simulink model "gm_uz_endat_interface_2025b"  (R2025b)
settings: Solver=FixedStepDiscrete  StartTime=0.0  StopTime=1.3e-3  RelTol=1e-3
undefined symbols (not defined in the file or in its folder): binary_or_gray, bit_sum, delay_first_clk_on_off, endat_clk_divider, endat_encoder_bit_width_multi_turn, endat_encoder_bit_width_single_turn, endat_encoder_number_of_CRC_bits, f_ADC, f_clock, PLL, t_ADC, t_clock, XData
libraries: hdlmdlgenlib x123, simulink x35, hdlsllib x29, simulink_extras x13
(part 2 of 4)

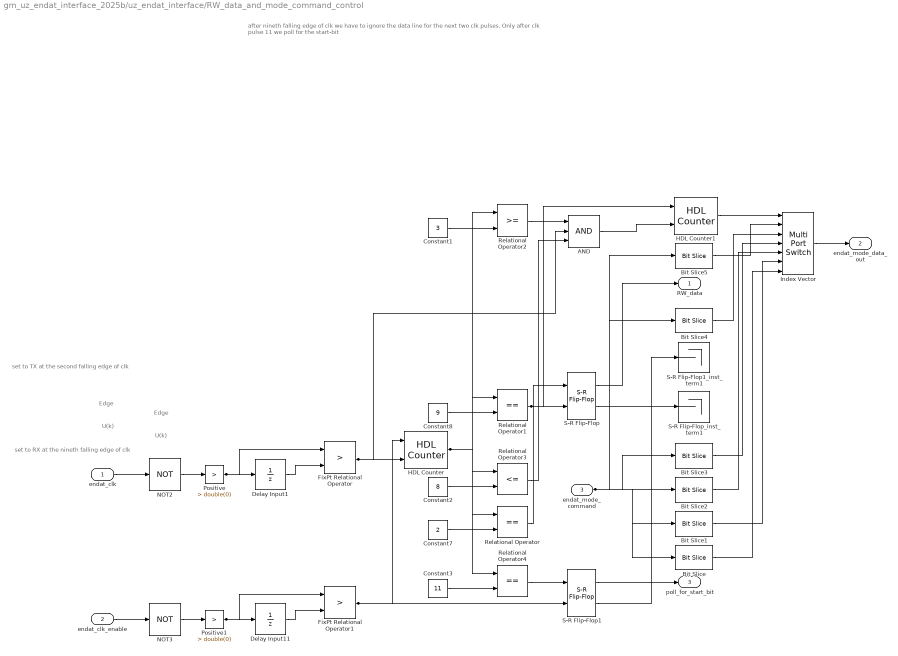
== system gm_uz_endat_interface_2025b/uz_endat_interface/RW_data_and_mode_command_control ==
  note: U(k)
  note: Edge
  note: U(k)
  note: Edge
  note: after nineth falling edge of clk we have to ignore the data line for the next two clk pulses. Only after clk pulse 11 we poll for the start-bit
  note: set to RX at the nineth falling edge of clk
  note: set to TX at the second falling edge of clk
  endat_clk : Inport  OutDataTypeStr=boolean  PortDimensions=1  SampleTime=1e-08
  endat_clk_enable : Inport  Port=2  OutDataTypeStr=boolean  PortDimensions=1  SampleTime=1e-08
  endat_mode_command : Inport  Port=3  OutDataTypeStr=uint32  PortDimensions=1  SampleTime=1e-08
  AND : Logic  Inputs=3  AllPortsSameDT=off  OutDataTypeStr=boolean  SampleTime=1e-08
  Bit Slice : hdlsllib/Logic and Bit Operations/Bit Slice  lidx=double(0)  ridx=double(0)
  Bit Slice1 : hdlsllib/Logic and Bit Operations/Bit Slice  lidx=double(1)  ridx=double(1)
  Bit Slice2 : hdlsllib/Logic and Bit Operations/Bit Slice  lidx=double(2)  ridx=double(2)
  Bit Slice3 : hdlsllib/Logic and Bit Operations/Bit Slice  lidx=double(3)  ridx=double(3)
  Bit Slice4 : hdlsllib/Logic and Bit Operations/Bit Slice  lidx=double(4)  ridx=double(4)
  Bit Slice5 : hdlsllib/Logic and Bit Operations/Bit Slice  lidx=double(5)  ridx=double(5)
  Constant1 : Constant  Value=3  OutDataTypeStr=uint8  SampleTime=1e-08
  Constant2 : Constant  Value=8  OutDataTypeStr=uint8  SampleTime=1e-08
  Constant3 : Constant  Value=11  OutDataTypeStr=uint8  SampleTime=1e-08
  Constant7 : Constant  Value=2  OutDataTypeStr=uint8  SampleTime=1e-08
  Constant8 : Constant  Value=9  OutDataTypeStr=uint8  SampleTime=1e-08
  Delay Input1 : UnitDelay  SampleTime=1e-08
  Delay Input11 : UnitDelay  SampleTime=1e-08
  FixPt Relational Operator : RelationalOperator  Operator=>  OutDataTypeStr=boolean  SampleTime=1e-08  InputSameDT=off
  FixPt Relational Operator1 : RelationalOperator  Operator=>  OutDataTypeStr=boolean  SampleTime=1e-08  InputSameDT=off
  HDL Counter : hdlsllib/Sources/HDL Counter  CountType=Free running  CountInit=0  CountStep=1  CountMax=25  CountFromType=Initial value  CountFrom=0  CountResetPort=on  CountLoadPort=off  CountEnbPort=on  CountDirPort=off  CountHitOutputPort=off  CountDataType=Unsigned  CountWordLen=8  CountFracLen=0  CountSampTime=1
  HDL Counter1 : hdlsllib/Sources/HDL Counter  CountType=Count limited  CountInit=0  CountStep=1  CountMax=5  CountFromType=Initial value  CountFrom=0  CountResetPort=on  CountLoadPort=off  CountEnbPort=on  CountDirPort=off  CountHitOutputPort=off  CountDataType=Unsigned  CountWordLen=8  CountFracLen=0  CountSampTime=1
  Index Vector : MultiPortSwitch  DataPortOrder=Zero-based contiguous  Inputs=6  DiagnosticForDefault=None  zeroidx=on  OutDataTypeStr=fixdt(0, 1, 0)  SampleTime=1e-08  SaturateOnIntegerOverflow=off  InputSameDT=off
  NOT2 : Logic  Operator=NOT  Inputs=1  AllPortsSameDT=off  OutDataTypeStr=boolean  SampleTime=1e-08
  NOT3 : Logic  Operator=NOT  Inputs=1  AllPortsSameDT=off  OutDataTypeStr=boolean  SampleTime=1e-08
  Positive : simulink/Logic and Bit Operations/Compare To Constant  relop=>  const=double(0)  OutDataTypeStr=boolean
  Positive1 : simulink/Logic and Bit Operations/Compare To Constant  relop=>  const=double(0)  OutDataTypeStr=boolean
  Relational Operator : RelationalOperator  Operator===  OutDataTypeStr=boolean  SampleTime=1e-08  InputSameDT=off
  Relational Operator1 : RelationalOperator  Operator===  OutDataTypeStr=boolean  SampleTime=1e-08  InputSameDT=off
  Relational Operator2 : RelationalOperator  OutDataTypeStr=boolean  SampleTime=1e-08  InputSameDT=off
  Relational Operator3 : RelationalOperator  Operator=<=  OutDataTypeStr=boolean  SampleTime=1e-08  InputSameDT=off
  Relational Operator4 : RelationalOperator  Operator===  OutDataTypeStr=boolean  SampleTime=1e-08  InputSameDT=off
  S-R Flip-Flop : simulink_extras/Flip Flops/S-R Flip-Flop  initial_condition=0
  S-R Flip-Flop1 : simulink_extras/Flip Flops/S-R Flip-Flop  initial_condition=0
  S-R Flip-Flop1_inst_term1 : Terminator
  S-R Flip-Flop_inst_term1 : Terminator
  RW_data : Outport  SampleTime=1e-08
  endat_mode_data_out : Outport  Port=2  SampleTime=1e-08
  poll_for_start_bit : Outport  Port=3  SampleTime=1e-08
  wires:
  endat_clk/1 -> NOT2/1
  Positive1/1 -> FixPt Relational Operator1/1, Delay Input11/1
  Bit Slice3/1 -> Index Vector/4
  endat_clk_enable/1 -> NOT3/1
  Delay Input1/1 -> FixPt Relational Operator/2
  NOT2/1 -> Positive/1
  Delay Input11/1 -> FixPt Relational Operator1/2
  NOT3/1 -> Positive1/1
  Positive/1 -> FixPt Relational Operator/1, Delay Input1/1
  FixPt Relational Operator/1 -> AND/2, HDL Counter/2
  FixPt Relational Operator1/1 -> S-R Flip-Flop1/2, HDL Counter/1
  Bit Slice4/1 -> Index Vector/3
  Constant1/1 -> Relational Operator2/2
  Constant7/1 -> Relational Operator/2
  Constant8/1 -> Relational Operator1/2
  HDL Counter/1 -> Relational Operator4/1, Relational Operator3/1, Relational Operator1/1, Relational Operator2/1, Relational Operator/1
  Constant3/1 -> Relational Operator4/2
  Constant2/1 -> Relational Operator3/2
  Relational Operator2/1 -> AND/1
  Relational Operator1/1 -> S-R Flip-Flop/2, HDL Counter1/1
  Relational Operator3/1 -> AND/3
  Relational Operator/1 -> S-R Flip-Flop/1
  Relational Operator4/1 -> S-R Flip-Flop1/1
  S-R Flip-Flop/2 -> S-R Flip-Flop_inst_term1/1
  S-R Flip-Flop/1 -> RW_data/1
  AND/1 -> HDL Counter1/2
  endat_mode_command/1 -> Bit Slice4/1, Bit Slice3/1, Bit Slice5/1, Bit Slice2/1, Bit Slice1/1, Bit Slice/1
  S-R Flip-Flop1/1 -> poll_for_start_bit/1
  S-R Flip-Flop1/2 -> S-R Flip-Flop1_inst_term1/1
  Index Vector/1 -> endat_mode_data_out/1
  HDL Counter1/1 -> Index Vector/1
  Bit Slice5/1 -> Index Vector/2
  Bit Slice2/1 -> Index Vector/5
  Bit Slice1/1 -> Index Vector/6
  Bit Slice/1 -> Index Vector/7

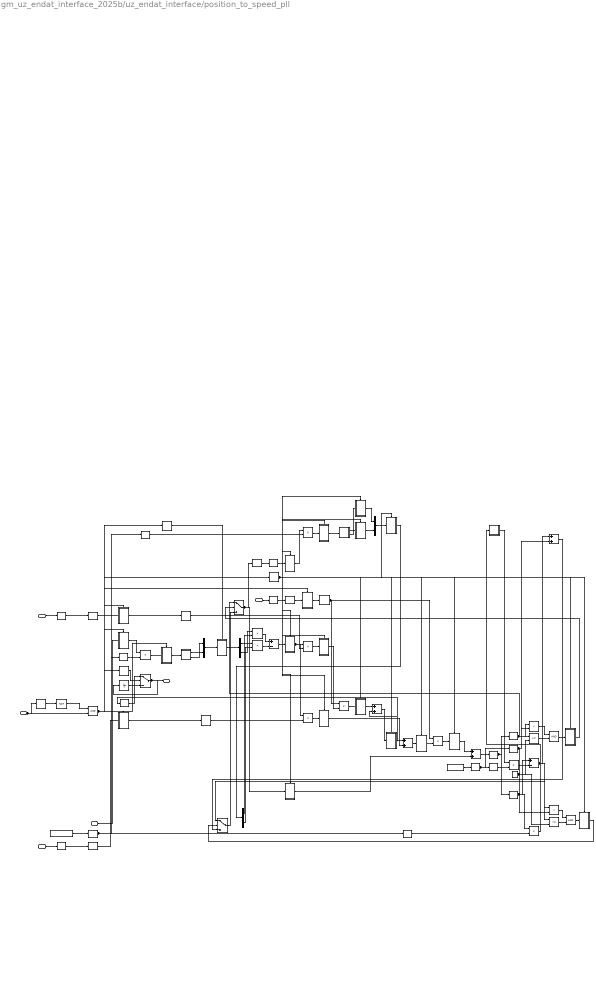
== system gm_uz_endat_interface_2025b/uz_endat_interface/position_to_speed_pll ==
  note: pi_controller
  note: +/- 198000
  note: -2 ... 2
  note: wrap 2pi
  note: <<1
  note: phase discriminator
  note: -1 ... 1
  note: pll
  note: -1 ... 1
  note: integrator
  note: 20
  note: +/- 1300
  note: remainder
  position_mech_SI : Inport  OutDataTypeStr=fixdt(0, 27, 24)  PortDimensions=1  SampleTime=1e-08
  t_sample : Inport  Port=2  OutDataTypeStr=fixdt(0, 18, 24)  PortDimensions=1  SampleTime=1e-08
  kp_pll : Inport  Port=3  OutDataTypeStr=fixdt(0, 18, 5)  PortDimensions=1  SampleTime=1e-08
  ki_pll : Inport  Port=4  OutDataTypeStr=fixdt(0, 18, 0)  PortDimensions=1  SampleTime=1e-08
  Trigger : Inport  Port=5  OutDataTypeStr=boolean  SampleTime=1e-08
  AND : Logic  AllPortsSameDT=off  OutDataTypeStr=boolean  SampleTime=1e-08
  AND1 : Logic  AllPortsSameDT=off  OutDataTypeStr=boolean  SampleTime=1e-08
  Constant1 : Constant  Value=0.1591548919677734375  OutDataTypeStr=fixdt(0, 18, 20)  SampleTime=1e-08
  Constant7 : Constant  Value=0  OutDataTypeStr=fixdt(0, 27, 24)  SampleTime=1e-08
  Constant8 : Constant  Value=6.283172607421875  OutDataTypeStr=fixdt(0, 18, 15)  SampleTime=1e-08
  Delay : Subsystem
      settings: MinAlgLoopOccurrences=on
  Delay1 : Subsystem
      settings: MinAlgLoopOccurrences=on
  Delay10 : Subsystem
      settings: MinAlgLoopOccurrences=on
  Delay11 : Subsystem
      settings: MinAlgLoopOccurrences=on
  Delay12 : Subsystem
      settings: MinAlgLoopOccurrences=on
  Delay13 : Subsystem
      settings: MinAlgLoopOccurrences=on
  Delay14 : Subsystem
      settings: MinAlgLoopOccurrences=on
  Delay18 : Subsystem
      settings: MinAlgLoopOccurrences=on
  Delay19 : Subsystem
      settings: MinAlgLoopOccurrences=on
  Delay2 : Subsystem
      settings: MinAlgLoopOccurrences=on
  Delay20 : Subsystem
      settings: MinAlgLoopOccurrences=on
  Delay21 : Subsystem
      settings: MinAlgLoopOccurrences=on
  Delay22 : Subsystem
      settings: MinAlgLoopOccurrences=on
  Delay23 : Subsystem
      settings: MinAlgLoopOccurrences=on
  Delay3 : Subsystem
      settings: MinAlgLoopOccurrences=on
  Delay4 : Subsystem
      settings: MinAlgLoopOccurrences=on
  Delay5 : Subsystem
      settings: MinAlgLoopOccurrences=on
  Delay6 : Subsystem
      settings: MinAlgLoopOccurrences=on
  Delay7 : Subsystem
      settings: MinAlgLoopOccurrences=on
  Delay8 : Subsystem
      settings: MinAlgLoopOccurrences=on
  Delay9 : Subsystem
      settings: MinAlgLoopOccurrences=on
  From{,1..6,11,13..15} (11 alike) : hdlmdlgenlib/Buffer
  Goto{,1..3,8,10..11} (7 alike) : hdlmdlgenlib/Buffer
  Product1 : Product  Inputs=**  OutDataTypeStr=fixdt(1, 27, 23)  SampleTime=1e-08
  Product10 : Product  Inputs=**  OutDataTypeStr=fixdt(1, 27, 20)  SampleTime=1e-08
  Product2 : Product  Inputs=**  OutDataTypeStr=fixdt(1, 27, 25)  SampleTime=1e-08
  Product3 : Product  Inputs=**  OutDataTypeStr=fixdt(1, 27, 25)  SampleTime=1e-08
  Product4 : Product  Inputs=**  OutDataTypeStr=fixdt(1, 27, 20)  SampleTime=1e-08
  Product5 : Product  Inputs=**  OutDataTypeStr=fixdt(1, 27, 8)  SampleTime=1e-08
  Product6 : Product  Inputs=**  OutDataTypeStr=fixdt(1, 27, 14)  SampleTime=1e-08
  Product7 : Product  Inputs=**  OutDataTypeStr=fixdt(1, 27, 23)  SampleTime=1e-08
  Product8 : Product  Inputs=**  OutDataTypeStr=fixdt(1, 27, 26)  SampleTime=1e-08
  Product9 : Product  Inputs=**  OutDataTypeStr=fixdt(1, 27, 20)  SampleTime=1e-08
  Relational Operator1 : RelationalOperator  Operator=<  OutDataTypeStr=boolean  SampleTime=1e-08  InputSameDT=off
  Relational Operator2 : RelationalOperator  OutDataTypeStr=boolean  SampleTime=1e-08  InputSameDT=off
  Relational Operator3 : RelationalOperator  Operator=<  OutDataTypeStr=boolean  SampleTime=1e-08  InputSameDT=off
  Relational Operator4 : RelationalOperator  OutDataTypeStr=boolean  SampleTime=1e-08  InputSameDT=off
  Sine HDL Optimized : Subsystem  mask(Sine and Cosine HDL optimized block){OutputFormula=sin(2*pi*u) and cos(2*pi*u), NumDataPoints=double(256), TableDataTypeStr=fixdt(0,26,20), SimulateLUTROMDelay=off}
      mask prompts: OutputFormula "Simulink:masks:OutputFormula_MP"; NumDataPoints "HDLShared:hdlshared:CosineHDL_Npts"; TableDataTypeStr "Simulink:blkprm_prompts:TABLE_UNIFIEDDATATYPE"; SimulateLUTROMDelay "HDLShared:hdlshared:CosineHDL_SimulateLUTDelay"
      mask help: Sine and Cosine HDL optimized block using quarter wave symmetry, and HDL friendly settings.
      mask init:
      | NumDataPoints = double(256);
      | OutputFormula = double(4);
      | SampleTime = double(-1);
      | SimulateLUTROMDelay = double(0);
      | TableDataTypeStr = fixdt(0,26,20);
      | curr_blk_name = 'uz_endat_interface_2025b/uz_endat_interface/position_to_speed_pll/Sine\nHDL Optimized';
      | sys_name = 'uz_endat_interface_2025b/uz_endat_interface/position_to_speed_pll';
      mask Help: helpview([docroot '/hdlcoder/helptargets.map'],'SineAndCosineHDL_Optimized');
      mask TypeOptions OutputFormula: sin(2*pi*u) | cos(2*pi*u) | exp(j*2*pi*u) | sin(2*pi*u) and cos(2*pi*u)
      mask Display:
      | port_label('input',1,'u')
      | port_label('output',1,'sin(2*pi*u)')
      | port_label('output',2,'cos(2*pi*u)')
      | xpos = 0.35;
      | yoffset = 0.5;
      | if ( SimulateLUTROMDelay )
      |   text(xpos,yoffset,'HDL (Z^{-1})','texmode','on')
      | else
      |    text(xpos,yoffset,'HDL')
      | end
  Sine HDL Optimized1 : Subsystem  mask(Sine and Cosine HDL optimized block){OutputFormula=sin(2*pi*u) and cos(2*pi*u), NumDataPoints=double(256), TableDataTypeStr=fixdt(0,26,20), SimulateLUTROMDelay=off}
      mask prompts: OutputFormula "Simulink:masks:OutputFormula_MP"; NumDataPoints "HDLShared:hdlshared:CosineHDL_Npts"; TableDataTypeStr "Simulink:blkprm_prompts:TABLE_UNIFIEDDATATYPE"; SimulateLUTROMDelay "HDLShared:hdlshared:CosineHDL_SimulateLUTDelay"
      mask help: Sine and Cosine HDL optimized block using quarter wave symmetry, and HDL friendly settings.
      mask init:
      | NumDataPoints = double(256);
      | OutputFormula = double(4);
      | SampleTime = double(-1);
      | SimulateLUTROMDelay = double(0);
      | TableDataTypeStr = fixdt(0,26,20);
      | curr_blk_name = 'uz_endat_interface_2025b/uz_endat_interface/position_to_speed_pll/Sine\nHDL Optimized1';
      | sys_name = 'uz_endat_interface_2025b/uz_endat_interface/position_to_speed_pll';
      mask Help: helpview([docroot '/hdlcoder/helptargets.map'],'SineAndCosineHDL_Optimized');
      mask TypeOptions OutputFormula: sin(2*pi*u) | cos(2*pi*u) | exp(j*2*pi*u) | sin(2*pi*u) and cos(2*pi*u)
      mask Display:
      | port_label('input',1,'u')
      | port_label('output',1,'sin(2*pi*u)')
      | port_label('output',2,'cos(2*pi*u)')
      | xpos = 0.35;
      | yoffset = 0.5;
      | if ( SimulateLUTROMDelay )
      |   text(xpos,yoffset,'HDL (Z^{-1})','texmode','on')
      | else
      |    text(xpos,yoffset,'HDL')
      | end
  Sum1 : Sum  Inputs=+-  OutDataTypeStr=fixdt(1, 27, 24)  AccumDataTypeStr=fixdt(1, 27, 24)  SampleTime=1e-08
  Sum2 : Sum  OutDataTypeStr=fixdt(1, 27, 16)  AccumDataTypeStr=fixdt(1, 32, 20)  SampleTime=1e-08
  Sum3 : Sum  OutDataTypeStr=fixdt(1, 27, 14)  AccumDataTypeStr=fixdt(1, 30, 16)  SampleTime=1e-08
  Sum4 : Sum  OutDataTypeStr=fixdt(1, 27, 23)  AccumDataTypeStr=fixdt(1, 31, 26)  SampleTime=1e-08
  Sum5 : Sum  Inputs=+-  OutDataTypeStr=fixdt(1, 27, 23)  AccumDataTypeStr=fixdt(1, 28, 23)  SampleTime=1e-08
  Sum6 : Sum  OutDataTypeStr=fixdt(1, 27, 23)  AccumDataTypeStr=fixdt(1, 28, 23)  SampleTime=1e-08
  Switch3 : Switch  Criteria=u2 > Threshold  Threshold="fi(0,0,1,0,\"hex\",\"0\")"  OutDataTypeStr=fixdt(1, 27, 23)  SampleTime=1e-08  SaturateOnIntegerOverflow=off  InputSameDT=off
  Switch4 : Switch  Criteria=u2 > Threshold  Threshold="fi(0,0,1,0,\"hex\",\"0\")"  OutDataTypeStr=fixdt(1, 27, 23)  SampleTime=1e-08  SaturateOnIntegerOverflow=off  InputSameDT=off
  Trigger_delay : Delay  DelayLength=double(1)  InitialCondition=0
  Trigger_delayed_inverted_and_Trigger : Logic  AllPortsSameDT=off  OutDataTypeStr=boolean  SampleTime=1e-08
  delayMatch{,1..5} (6 alike) : Delay  DelayLength=double(1)  InitialCondition=0
  fixed_point_floor : Subsystem
  mux : Mux  Inputs=2
  mux1 : Mux  Inputs=2
  not_Trigger_delayed : Logic  Operator=NOT  Inputs=1  AllPortsSameDT=off  OutDataTypeStr=boolean  SampleTime=1e-08
  omega_mechbypassMux : Switch  Criteria=u2 ~= 0  Threshold=double(0)  OutDataTypeStr=fixdt(1, 27, 16)  SampleTime=1e-08  SaturateOnIntegerOverflow=off  InputSameDT=off
  out0_bypass : UnitDelay  InitialCondition="fi(0,1,27,16,\"hex\",\"0000000\")"  SampleTime=1e-08
  t : Demux  Outputs=2
  t1 : Demux  Outputs=2
  t2 : hdlmdlgenlib/Buffer
  speed_mech_SI : Outport  SampleTime=1e-08  InitialOutput=[0]
  wires:
  Product5/1 -> Delay5/1(in0)
  delayMatch1/1 -> Delay2/Enable, Delay11/Enable, Delay9/Enable, Delay18/Enable, Delay5/Enable, Delay3/Enable, Delay21/Enable, Delay20/Enable, Delay12/Enable, Delay10/Enable, Delay/Enable, Delay4/Enable, Delay23/Enable, Delay19/Enable, Delay22/Enable
  Trigger/1 -> Trigger_delayed_inverted_and_Trigger/2, Trigger_delay/1
  Goto10/1 -> From15/1, From11/1
  Goto3/1 -> From5/1, From4/1, From6/1
  ki_pll/1 -> Goto2/1
  Goto1/1 -> From1/1
  Constant1/1 -> Goto3/1
  Trigger_delay/1 -> not_Trigger_delayed/1
  t_sample/1 -> Goto/1
  Sine HDL Optimized/2(y) -> Delay23/1(in0)
  delayMatch3/1 -> Product8/1, Product4/1
  Product6/1 -> Delay3/1(in0)
  Goto8/1 -> From3/1
  Delay6/1(out0) -> delayMatch3/1
  kp_pll/1 -> Goto1/1
  Delay11/1(out0) -> Product9/1
  Switch3/1 -> Goto8/1, Delay19/1(in0)
  omega_mechbypassMux/1 -> out0_bypass/1, speed_mech_SI/1
  Goto2/1 -> From2/1
  Product4/1 -> Delay4/1(in0)
  not_Trigger_delayed/1 -> Trigger_delayed_inverted_and_Trigger/1
  Delay12/1(out0) -> Sine HDL Optimized/1(u)
  From2/1 -> Delay7/1(in0)
  Goto/1 -> From/1
  Trigger_delayed_inverted_and_Trigger/1 -> Delay7/Enable, delayMatch1/1, Delay14/Enable, Delay13/Enable, Delay8/Enable, delayMatch/1, delayMatch5/1, Delay6/Enable
  position_mech_SI/1 -> Delay13/1(in0)
  From3/1 -> Delay11/1(in0)
  From1/1 -> Delay8/1(in0)
  Delay7/1(out0) -> delayMatch4/1
  Delay14/1(out0) -> Sine HDL Optimized1/1(u)
  Sine HDL Optimized1/1(x) -> mux/2
  Delay13/1(out0) -> Product10/1
  From6/1 -> Product10/2
  Delay1/1(out0) -> t/1
  delayMatch5/1 -> omega_mechbypassMux/2
  out0_bypass/1 -> omega_mechbypassMux/3
  t2/1 -> omega_mechbypassMux/1
  Delay8/1(out0) -> delayMatch2/1
  From5/1 -> Product9/2
  Product10/1 -> Delay14/1(in0)
  Delay4/1(out0) -> Sum2/1
  delayMatch/1 -> Delay1/Enable
  From15/1 -> Product7/1, Sum5/1
  Sine HDL Optimized/1(x) -> Delay22/1(in0)
  Sum1/1 -> Delay2/1(in0)
  delayMatch4/1 -> Product5/2
  Sine HDL Optimized1/2(y) -> mux/1
  From/1 -> Delay6/1(in0)
  Product2/1 -> Sum1/2
  mux/1 -> Delay1/1(in0)
  delayMatch2/1 -> Product6/2
  Switch4/1 -> Switch3/3
  Sum4/1 -> Goto10/1
  t/2 -> Product3/1
  t/1 -> Product2/1
  t1/2 -> Product2/2
  t1/1 -> Product3/2
  Product3/1 -> Sum1/1
  Delay2/1(out0) -> Product6/1, Product5/1
  AND1/1 -> Delay20/1(in0)
  Delay19/1(out0) -> Sum4/2
  Product9/1 -> Delay12/1(in0)
  Delay5/1(out0) -> Product4/2
  Delay3/1(out0) -> Sum3/2
  Delay23/1(out0) -> mux1/1
  Delay22/1(out0) -> mux1/2
  mux1/1 -> Delay18/1(in0)
  Sum2/1 -> Delay/1(in0)
  Delay18/1(out0) -> t1/1
  Delay/1(out0) -> t2/1, Sum2/2, Sum3/1
  Sum3/1 -> Delay9/1(in0)
  From4/1 -> Product7/2
  Delay9/1(out0) -> Product8/2
  Product8/1 -> Delay10/1(in0)
  From14/1 -> Product1/2
  Delay10/1(out0) -> Sum4/1
  Constant8/1 -> Goto11/1
  Goto11/1 -> From13/1, From14/1
  fixed_point_floor/1(y) -> Product1/1
  From11/1 -> Switch3/1, Relational Operator2/1, Relational Operator1/1
  From13/1 -> Relational Operator3/2, Sum6/2, Relational Operator1/2
  Product1/1 -> Sum5/2
  Constant7/1 -> Relational Operator4/2, Relational Operator2/2
  Relational Operator1/1 -> AND/1
  Relational Operator2/1 -> AND/2
  Sum5/1 -> Switch4/1, Sum6/1, Relational Operator4/1, Relational Operator3/1
  Product7/1 -> fixed_point_floor/1(x)
  Sum6/1 -> Switch4/3
  AND/1 -> Delay21/1(in0)
  Delay20/1(out0) -> Switch4/2
  Relational Operator3/1 -> AND1/1
  Relational Operator4/1 -> AND1/2
  Delay21/1(out0) -> Switch3/2

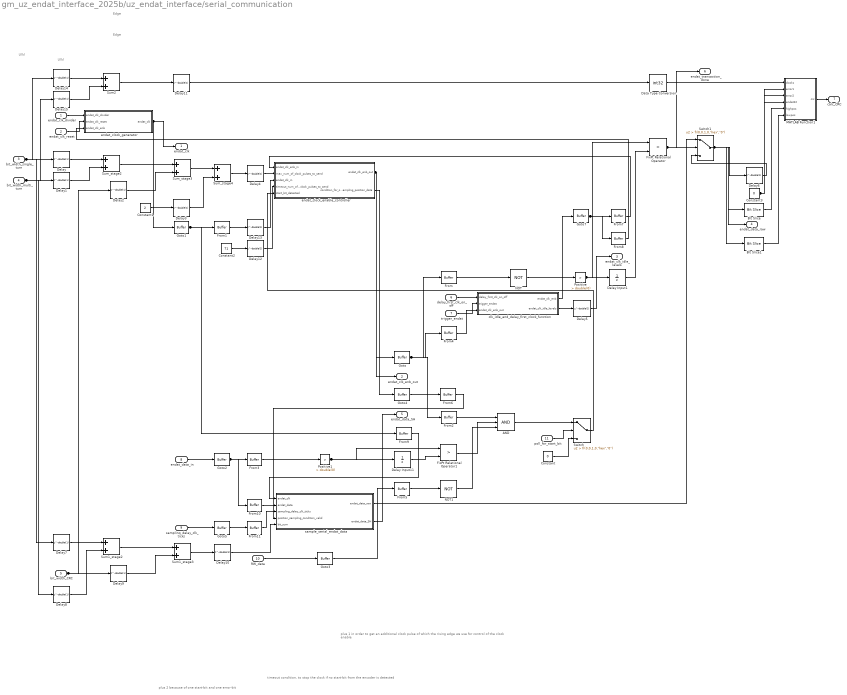
== system gm_uz_endat_interface_2025b/uz_endat_interface/serial_communication ==
  note: U(k)
  note: Edge
  note: U(k)
  note: Edge
  note: plus 1 in order to get an additional clock pulse of which the rising edge we use for control of the clock enable
  note: timeout condition, to stop the clock if no start-bit from the encoder is detected
  note: plus 2 because of one start-bit and one error-bit
  endat_clk_divider : Inport  OutDataTypeStr=uint32  PortDimensions=1  SampleTime=1e-08
  endat_clk_reset : Inport  Port=2  OutDataTypeStr=boolean  PortDimensions=1  SampleTime=1e-08
  bit_width_single_turn : Inport  Port=3  OutDataTypeStr=uint32  PortDimensions=1  SampleTime=1e-08
  bit_width_multi_turn : Inport  Port=4  OutDataTypeStr=uint32  PortDimensions=1  SampleTime=1e-08
  bit_width_CRC : Inport  Port=5  OutDataTypeStr=uint32  PortDimensions=1  SampleTime=1e-08
  delay_first_clk_on_off : Inport  Port=6  OutDataTypeStr=boolean  PortDimensions=1  SampleTime=1e-08
  trigger_endat : Inport  Port=7  OutDataTypeStr=boolean  PortDimensions=1  SampleTime=1e-08
  endat_data_in : Inport  Port=8  OutDataTypeStr=boolean  PortDimensions=1  SampleTime=1e-08
  sampling_delay_clk_ticks : Inport  Port=9  OutDataTypeStr=uint32  PortDimensions=1  SampleTime=1e-08
  RW_data : Inport  Port=10  OutDataTypeStr=boolean  PortDimensions=1  SampleTime=1e-08
  poll_for_start_bit : Inport  Port=11  OutDataTypeStr=boolean  PortDimensions=1  SampleTime=1e-08
  AND : Logic  Inputs=3  AllPortsSameDT=off  OutDataTypeStr=boolean  SampleTime=1e-08
  Bit Slice : hdlsllib/Logic and Bit Operations/Bit Slice  lidx=double(63)  ridx=double(32)
  Bit Slice1 : hdlsllib/Logic and Bit Operations/Bit Slice  lidx=double(31)  ridx=double(0)
  Constant : Constant  Value=0  OutDataTypeStr=boolean  SampleTime=1e-08
  Constant1 : Constant  Value=2  OutDataTypeStr=uint32  SampleTime=1e-08
  Constant2 : Constant  Value=71  OutDataTypeStr=uint32  SampleTime=1e-08
  Constant3 : Constant  Value=0  OutDataTypeStr=uint32  SampleTime=1e-08
  Data Type Conversion : DataTypeConversion  OutDataTypeStr=int32  SampleTime=1e-08  SaturateOnIntegerOverflow=off  RndMeth=Floor
  Delay{,1..15} (16 alike) : Delay  DelayLength=double(1)  InitialCondition=0  SampleTime=1e-08
  Delay Input1 : UnitDelay  SampleTime=1e-08
  Delay Input11 : UnitDelay  SampleTime=1e-08
  FixPt Relational Operator : RelationalOperator  Operator=>  OutDataTypeStr=boolean  SampleTime=1e-08  InputSameDT=off
  FixPt Relational Operator1 : RelationalOperator  Operator=>  OutDataTypeStr=boolean  SampleTime=1e-08  InputSameDT=off
  From{,1..11} (12 alike) : hdlmdlgenlib/Buffer
  Goto{,1..5,7} (7 alike) : hdlmdlgenlib/Buffer
  MATLAB Function1 : Subsystem
  NOT : Logic  Operator=NOT  Inputs=1  AllPortsSameDT=off  OutDataTypeStr=boolean  SampleTime=1e-08
  NOT1 : Logic  Operator=NOT  Inputs=1  AllPortsSameDT=off  OutDataTypeStr=boolean  SampleTime=1e-08
  Positive : simulink/Logic and Bit Operations/Compare To Constant  relop=>  const=double(0)  OutDataTypeStr=boolean
  Positive1 : simulink/Logic and Bit Operations/Compare To Constant  relop=>  const=double(0)  OutDataTypeStr=boolean
  Sum1_stage2 : Sum  OutDataTypeStr=fixdt(0, 33, 0)  AccumDataTypeStr=uint32  SampleTime=1e-08
  Sum1_stage3 : Sum  OutDataTypeStr=uint32  AccumDataTypeStr=uint32  SampleTime=1e-08
  Sum2 : Sum  OutDataTypeStr=uint32  AccumDataTypeStr=uint32  SampleTime=1e-08
  Sum_stage2 : Sum  OutDataTypeStr=fixdt(0, 33, 0)  AccumDataTypeStr=uint32  SampleTime=1e-08
  Sum_stage3 : Sum  OutDataTypeStr=fixdt(0, 34, 0)  AccumDataTypeStr=uint32  SampleTime=1e-08
  Sum_stage4 : Sum  OutDataTypeStr=uint32  AccumDataTypeStr=uint32  SampleTime=1e-08
  Switch : Switch  Criteria=u2 > Threshold  Threshold="fi(0,0,1,0,\"hex\",\"0\")"  OutDataTypeStr=boolean  SampleTime=1e-08  SaturateOnIntegerOverflow=off  InputSameDT=off
  Switch1 : Switch  Criteria=u2 > Threshold  Threshold="fi(0,0,1,0,\"hex\",\"0\")"  OutDataTypeStr=fixdt(0, 64, 0)  SampleTime=1e-08  SaturateOnIntegerOverflow=off  InputSameDT=off
  clk_idle_and_delay_first_clock_function : Subsystem
  endat_clock_enable_controller : Subsystem
  endat_clock_generator : Subsystem
  sample_serial_endat_data : Subsystem
  endat_clk : Outport  SampleTime=1e-08
  endat_clk_enb_out : Outport  Port=2  SampleTime=1e-08
  endat_clk_idle_levels : Outport  Port=3  SampleTime=1e-08
  endat_data_raw : Outport  Port=4  SampleTime=1e-08
  endat_data_SH : Outport  Port=5  SampleTime=1e-08
  endat_transaction_done : Outport  Port=6  SampleTime=1e-08
  calc_CRC : Outport  Port=7  SampleTime=1e-08
  wires:
  NOT/1 -> Positive/1
  endat_clk_divider/1 -> endat_clock_generator/1(endat_clk_divider)
  bit_width_single_turn/1 -> Delay7/1, Delay/1, Delay14/1
  bit_width_multi_turn/1 -> Delay8/1, Delay1/1, Delay15/1
  poll_for_start_bit/1 -> Switch/2
  Delay14/1 -> Sum2/1
  Delay15/1 -> Sum2/2
  endat_clk_reset/1 -> endat_clock_generator/2(endat_clk_reset)
  Delay/1 -> Sum_stage2/1
  Delay10/1 -> sample_serial_endat_data/5(bit_sum)
  Delay1/1 -> Sum_stage2/2
  Delay7/1 -> Sum1_stage2/1
  bit_width_CRC/1 -> Delay9/1, Delay2/1
  Delay8/1 -> Sum1_stage2/2
  Goto3/1 -> From5/1
  Sum2/1 -> Delay11/1
  endat_clock_generator/1(endat_clk) -> endat_clk/1, Goto1/1
  Sum_stage2/1 -> Sum_stage3/1
  endat_data_in/1 -> Goto2/1
  Delay2/1 -> Sum_stage3/2
  Constant/1 -> Switch/3
  Delay9/1 -> Sum1_stage3/2
  Constant1/1 -> Delay3/1
  Goto4/1 -> From6/1
  Sum1_stage2/1 -> Sum1_stage3/1
  Delay11/1 -> Data Type Conversion/1
  From11/1 -> sample_serial_endat_data/3(sampling_delay_clk_ticks)
  Sum_stage3/1 -> Sum_stage4/1
  Delay3/1 -> Sum_stage4/2
  From/1 -> NOT/1
  Goto1/1 -> From9/1, From1/1
  Delay13/1 -> endat_clock_enable_controller/3(endat_clk_in)
  sampling_delay_clk_ticks/1 -> Goto5/1
  Sum1_stage3/1 -> Delay10/1
  clk_idle_and_delay_first_clock_function/1(endat_clk_enb) -> Goto7/1
  Sum_stage4/1 -> Delay4/1
  From1/1 -> Delay13/1
  FixPt Relational Operator1/1 -> AND/2
  Delay4/1 -> endat_clock_enable_controller/2(max_num_of_clock_pulses_to_send)
  Constant2/1 -> Delay12/1
  Goto2/1 -> From10/1, From3/1
  Goto5/1 -> From11/1
  Delay12/1 -> endat_clock_enable_controller/4(timeout_num_of_clock_pulses_to_send)
  NOT1/1 -> AND/3
  From3/1 -> Positive1/1
  From10/1 -> sample_serial_endat_data/2(endat_data)
  endat_clock_enable_controller/2(condition_for_start_sampling_position_data) -> Goto4/1
  RW_data/1 -> Goto3/1
  endat_clock_enable_controller/1(endat_clk_enb_out) -> endat_clk_enb_out/1, Goto/1
  Positive1/1 -> FixPt Relational Operator1/1, Delay Input11/1
  sample_serial_endat_data/1(endat_data_raw) -> Switch1/1
  clk_idle_and_delay_first_clock_function/2(endat_clk_idle_levels) -> Delay5/1
  sample_serial_endat_data/2(endat_data_SH) -> endat_data_SH/1
  Goto7/1 -> From8/1, From7/1
  Goto/1 -> From/1, From4/1, From2/1
  From9/1 -> sample_serial_endat_data/1(endat_clk)
  Delay Input11/1 -> FixPt Relational Operator1/2
  From5/1 -> NOT1/1
  delay_first_clk_on_off/1 -> clk_idle_and_delay_first_clock_function/1(delay_first_clk_on_off)
  trigger_endat/1 -> clk_idle_and_delay_first_clock_function/2(trigger_endat)
  From4/1 -> clk_idle_and_delay_first_clock_function/3(endat_clk_enb_out)
  From6/1 -> sample_serial_endat_data/4(position_sampling_condition_valid)
  From2/1 -> AND/1
  AND/1 -> Switch/1
  Positive/1 -> FixPt Relational Operator/1, Delay Input1/1
  Delay5/1 -> endat_clk_idle_levels/1
  Switch/1 -> endat_clock_enable_controller/5(start_bit_detected)
  From7/1 -> endat_clock_enable_controller/1(endat_clk_enb_in)
  From8/1 -> endat_clock_generator/3(endat_clk_enb)
  Delay Input1/1 -> FixPt Relational Operator/2
  Data Type Conversion/1 -> MATLAB Function1/1(clocks)
  FixPt Relational Operator/1 -> endat_transaction_done/1, Switch1/2
  Switch1/1 -> Bit Slice1/1, Delay6/1, endat_data_raw/1, Bit Slice/1
  Delay6/1 -> Switch1/3
  Constant3/1 -> MATLAB Function1/4(endat22), MATLAB Function1/3(error2), MATLAB Function1/2(error1)
  Bit Slice/1 -> MATLAB Function1/5(highpos)
  Bit Slice1/1 -> MATLAB Function1/6(lowpos)
  MATLAB Function1/1(crc) -> calc_CRC/1

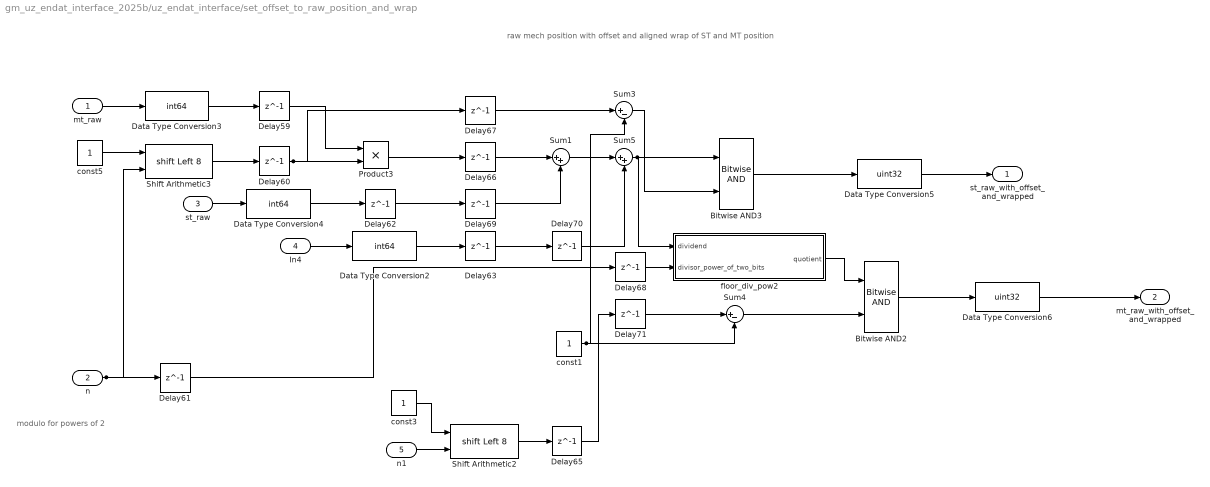
== system gm_uz_endat_interface_2025b/uz_endat_interface/set_offset_to_raw_position_and_wrap ==
  note: modulo for powers of 2
  note: raw mech position with offset and aligned wrap of ST and MT position
  mt_raw : Inport  OutDataTypeStr=uint32  PortDimensions=1  SampleTime=1e-08
  n : Inport  Port=2  OutDataTypeStr=uint32  PortDimensions=1  SampleTime=1e-08
  st_raw : Inport  Port=3  OutDataTypeStr=uint32  PortDimensions=1  SampleTime=1e-08
  In4 : Inport  Port=4  OutDataTypeStr=int32  PortDimensions=1  SampleTime=1e-08
  n1 : Inport  Port=5  OutDataTypeStr=uint32  PortDimensions=1  SampleTime=1e-08
  Bitwise AND2 : simulink/Logic and Bit Operations/Bitwise Operator  logicop=AND  UseBitMask=off  NumInputPorts=2  BitMask=bin2dec('11011001')  BitMaskRealWorld=Stored Integer
      settings: LibrarySourceBlock=|
      | simulink/Quick Insert/Logic and Bit
      | Operations/Bitwise AND
  Bitwise AND3 : simulink/Logic and Bit Operations/Bitwise Operator  logicop=AND  UseBitMask=off  NumInputPorts=2  BitMask=bin2dec('11011001')  BitMaskRealWorld=Stored Integer
      settings: LibrarySourceBlock=|
      | simulink/Quick Insert/Logic and Bit
      | Operations/Bitwise AND
  Data Type Conversion2 : DataTypeConversion  OutDataTypeStr=int64  SaturateOnIntegerOverflow=off  RndMeth=Floor
  Data Type Conversion3 : DataTypeConversion  OutDataTypeStr=int64  SaturateOnIntegerOverflow=off  RndMeth=Floor
  Data Type Conversion4 : DataTypeConversion  OutDataTypeStr=int64  SaturateOnIntegerOverflow=off  RndMeth=Floor
  Data Type Conversion5 : DataTypeConversion  OutDataTypeStr=uint32  SaturateOnIntegerOverflow=off  RndMeth=Floor
  Data Type Conversion6 : DataTypeConversion  OutDataTypeStr=uint32  SaturateOnIntegerOverflow=off  RndMeth=Floor
  Delay{59..63,65..71} (12 alike) : Delay  DelayLength=1  InitialCondition=0
  Product3 : Product  OutDataTypeStr=int64
  Shift Arithmetic2 : ArithShift  BitShiftNumberSource=Input port  BitShiftNumber=8  BitShiftDirection=Left
      settings: InputPortMap=u0,p1
  Shift Arithmetic3 : ArithShift  BitShiftNumberSource=Input port  BitShiftNumber=8  BitShiftDirection=Left
      settings: InputPortMap=u0,p1
  Sum1 : Sum  Inputs=|++  OutDataTypeStr=int64
  Sum3 : Sum  Inputs=|+-  OutDataTypeStr=int64
  Sum4 : Sum  Inputs=|+-  OutDataTypeStr=int64
  Sum5 : Sum  Inputs=|++  OutDataTypeStr=int64
  const1 : Constant  OutDataTypeStr=int64  SampleTime=t_clock
  const3 : Constant  OutDataTypeStr=int64  SampleTime=t_clock
  const5 : Constant  OutDataTypeStr=int64  SampleTime=t_clock
  floor_div_pow2 : Subsystem
  st_raw_with_offset_and_wrapped : Outport  SampleTime=1e-08
  mt_raw_with_offset_and_wrapped : Outport  Port=2  SampleTime=1e-08
  wires:
  const3/1 -> Shift Arithmetic2/1
  mt_raw/1 -> Data Type Conversion3/1
  Shift Arithmetic3/1 -> Delay60/1
  const5/1 -> Shift Arithmetic3/1
  Delay65/1 -> Delay71/1
  n/1 -> Shift Arithmetic3/2, Delay61/1
  Data Type Conversion3/1 -> Delay59/1
  Data Type Conversion2/1 -> Delay63/1
  st_raw/1 -> Data Type Conversion4/1
  Delay61/1 -> Delay68/1
  Delay59/1 -> Product3/1
  Delay60/1 -> Delay67/1, Product3/2
  Data Type Conversion4/1 -> Delay62/1
  Bitwise AND3/1 -> Data Type Conversion5/1
  In4/1 -> Data Type Conversion2/1
  Product3/1 -> Delay66/1
  Delay62/1 -> Delay69/1
  n1/1 -> Shift Arithmetic2/2
  Delay67/1 -> Sum3/1
  Delay66/1 -> Sum1/1
  Delay69/1 -> Sum1/2
  Data Type Conversion6/1 -> mt_raw_with_offset_and_wrapped/1
  Delay63/1 -> Delay70/1
  Sum3/1 -> Bitwise AND3/2
  Shift Arithmetic2/1 -> Delay65/1
  Sum1/1 -> Sum5/1
  Delay70/1 -> Sum5/2
  const1/1 -> Sum4/2, Sum3/2
  Sum5/1 -> floor_div_pow2/1(dividend), Bitwise AND3/1
  Delay68/1 -> floor_div_pow2/2(divisor_power_of_two_bits)
  Delay71/1 -> Sum4/1
  floor_div_pow2/1(quotient) -> Bitwise AND2/1
  Sum4/1 -> Bitwise AND2/2
  Data Type Conversion5/1 -> st_raw_with_offset_and_wrapped/1
  Bitwise AND2/1 -> Data Type Conversion6/1

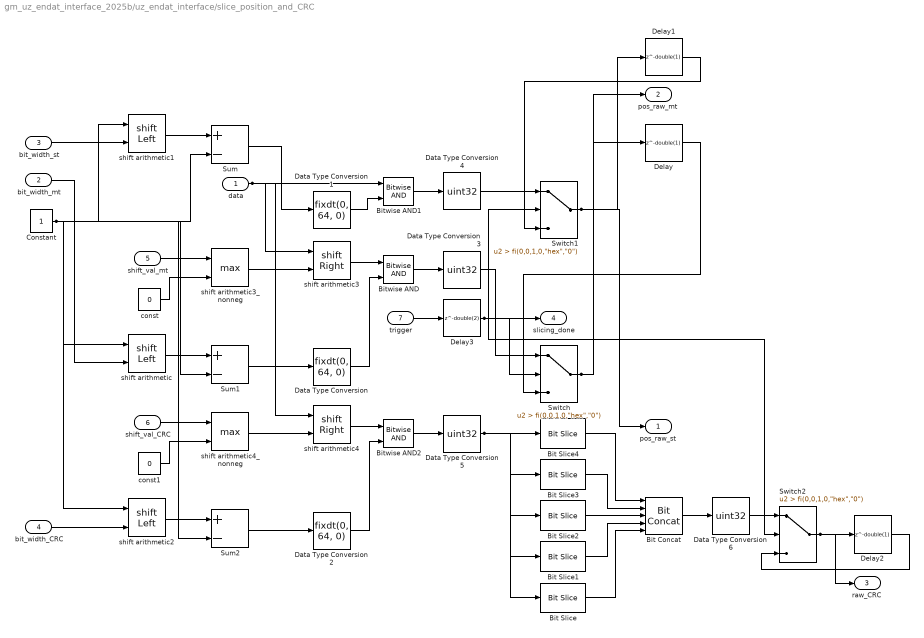
== system gm_uz_endat_interface_2025b/uz_endat_interface/slice_position_and_CRC ==
  data : Inport  OutDataTypeStr=fixdt(0, 64, 0)  PortDimensions=1  SampleTime=1e-08
  bit_width_mt : Inport  Port=2  OutDataTypeStr=uint32  PortDimensions=1  SampleTime=1e-08
  bit_width_st : Inport  Port=3  OutDataTypeStr=uint32  PortDimensions=1  SampleTime=1e-08
  bit_width_CRC : Inport  Port=4  OutDataTypeStr=uint32  PortDimensions=1  SampleTime=1e-08
  shift_val_mt : Inport  Port=5  OutDataTypeStr=int32  PortDimensions=1  SampleTime=1e-08
  shift_val_CRC : Inport  Port=6  OutDataTypeStr=int32  PortDimensions=1  SampleTime=1e-08
  trigger : Inport  Port=7  OutDataTypeStr=boolean  PortDimensions=1  SampleTime=1e-08
  Bit Concat : hdlsllib/Logic and Bit Operations/Bit Concat  numInputs=5
  Bit Slice : hdlsllib/Logic and Bit Operations/Bit Slice  lidx=double(4)  ridx=double(4)
  Bit Slice1 : hdlsllib/Logic and Bit Operations/Bit Slice  lidx=double(3)  ridx=double(3)
  Bit Slice2 : hdlsllib/Logic and Bit Operations/Bit Slice  lidx=double(2)  ridx=double(2)
  Bit Slice3 : hdlsllib/Logic and Bit Operations/Bit Slice  lidx=double(1)  ridx=double(1)
  Bit Slice4 : hdlsllib/Logic and Bit Operations/Bit Slice  lidx=double(0)  ridx=double(0)
  Bitwise AND : simulink/Logic and Bit Operations/Bitwise Operator  logicop=AND  UseBitMask=off  NumInputPorts=2  BitMask=double(0)  BitMaskRealWorld=Real World Value
  Bitwise AND1 : simulink/Logic and Bit Operations/Bitwise Operator  logicop=AND  UseBitMask=off  NumInputPorts=2  BitMask=double(0)  BitMaskRealWorld=Real World Value
  Bitwise AND2 : simulink/Logic and Bit Operations/Bitwise Operator  logicop=AND  UseBitMask=off  NumInputPorts=2  BitMask=double(0)  BitMaskRealWorld=Real World Value
  Constant : Constant  OutDataTypeStr=uint32  SampleTime=1e-08
  Data Type Conversion : DataTypeConversion  OutDataTypeStr=fixdt(0, 64, 0)  SampleTime=1e-08  SaturateOnIntegerOverflow=off  RndMeth=Floor
  Data Type Conversion1 : DataTypeConversion  OutDataTypeStr=fixdt(0, 64, 0)  SampleTime=1e-08  SaturateOnIntegerOverflow=off  RndMeth=Floor
  Data Type Conversion2 : DataTypeConversion  OutDataTypeStr=fixdt(0, 64, 0)  SampleTime=1e-08  SaturateOnIntegerOverflow=off  RndMeth=Floor
  Data Type Conversion{3..6} (4 alike) : DataTypeConversion  OutDataTypeStr=uint32  SampleTime=1e-08  SaturateOnIntegerOverflow=off  RndMeth=Floor
  Delay : Delay  DelayLength=double(1)  InitialCondition=0  SampleTime=1e-08
  Delay1 : Delay  DelayLength=double(1)  InitialCondition=0  SampleTime=1e-08
  Delay2 : Delay  DelayLength=double(1)  InitialCondition=0  SampleTime=1e-08
  Delay3 : Delay  DelayLength=double(2)  InitialCondition=0  SampleTime=1e-08
  Sum : Sum  Inputs=+-  OutDataTypeStr=uint32  AccumDataTypeStr=uint32  SampleTime=1e-08
  Sum1 : Sum  Inputs=+-  OutDataTypeStr=uint32  AccumDataTypeStr=uint32  SampleTime=1e-08
  Sum2 : Sum  Inputs=+-  OutDataTypeStr=uint32  AccumDataTypeStr=uint32  SampleTime=1e-08
  Switch : Switch  Criteria=u2 > Threshold  Threshold="fi(0,0,1,0,\"hex\",\"0\")"  OutDataTypeStr=uint32  SampleTime=1e-08  SaturateOnIntegerOverflow=off  InputSameDT=off
  Switch1 : Switch  Criteria=u2 > Threshold  Threshold="fi(0,0,1,0,\"hex\",\"0\")"  OutDataTypeStr=uint32  SampleTime=1e-08  SaturateOnIntegerOverflow=off  InputSameDT=off
  Switch2 : Switch  Criteria=u2 > Threshold  Threshold="fi(0,0,1,0,\"hex\",\"0\")"  OutDataTypeStr=uint32  SampleTime=1e-08  SaturateOnIntegerOverflow=off  InputSameDT=off
  const : Constant  Value=0  OutDataTypeStr=int32  SampleTime=1e-08
  const1 : Constant  Value=0  OutDataTypeStr=int32  SampleTime=1e-08
  shift arithmetic : ArithShift  BitShiftNumberSource=Input port  BitShiftDirection=Left
      settings: InputPortMap=u0,p1
  shift arithmetic1 : ArithShift  BitShiftNumberSource=Input port  BitShiftDirection=Left
      settings: InputPortMap=u0,p1
  shift arithmetic2 : ArithShift  BitShiftNumberSource=Input port  BitShiftDirection=Left
      settings: InputPortMap=u0,p1
  shift arithmetic3 : ArithShift  BitShiftNumberSource=Input port  BitShiftDirection=Right
      settings: InputPortMap=u0,p1
  shift arithmetic3_nonneg : MinMax  Function=max  Inputs=2
  shift arithmetic4 : ArithShift  BitShiftNumberSource=Input port  BitShiftDirection=Right
      settings: InputPortMap=u0,p1
  shift arithmetic4_nonneg : MinMax  Function=max  Inputs=2
  pos_raw_st : Outport  SampleTime=1e-08
  pos_raw_mt : Outport  Port=2  SampleTime=1e-08
  raw_CRC : Outport  Port=3  SampleTime=1e-08
  slicing_done : Outport  Port=4  SampleTime=1e-08
  wires:
  Bit Slice1/1 -> Bit Concat/4
  bit_width_st/1 -> shift arithmetic1/2
  bit_width_mt/1 -> shift arithmetic/2
  const/1 -> shift arithmetic3_nonneg/2
  bit_width_CRC/1 -> shift arithmetic2/2
  Constant/1 -> Sum2/2, Sum1/2, Sum/2, shift arithmetic2/1, shift arithmetic1/1, shift arithmetic/1
  shift arithmetic1/1 -> Sum/1
  Bit Slice/1 -> Bit Concat/5
  shift arithmetic/1 -> Sum1/1
  shift_val_mt/1 -> shift arithmetic3_nonneg/1
  Sum2/1 -> Data Type Conversion2/1
  shift_val_CRC/1 -> shift arithmetic4_nonneg/1
  const1/1 -> shift arithmetic4_nonneg/2
  Bit Slice4/1 -> Bit Concat/1
  shift arithmetic2/1 -> Sum2/1
  Sum/1 -> Data Type Conversion1/1
  data/1 -> Bitwise AND1/1, shift arithmetic4/1, shift arithmetic3/1
  trigger/1 -> Delay3/1
  shift arithmetic3_nonneg/1 -> shift arithmetic3/2
  Sum1/1 -> Data Type Conversion/1
  shift arithmetic4_nonneg/1 -> shift arithmetic4/2
  Switch1/1 -> pos_raw_st/1, Delay1/1
  Data Type Conversion1/1 -> Bitwise AND1/2
  shift arithmetic3/1 -> Bitwise AND/1
  Data Type Conversion/1 -> Bitwise AND/2
  shift arithmetic4/1 -> Bitwise AND2/1
  Delay1/1 -> Switch1/3
  Data Type Conversion2/1 -> Bitwise AND2/2
  Bitwise AND1/1 -> Data Type Conversion4/1
  Bitwise AND/1 -> Data Type Conversion3/1
  Bit Concat/1 -> Data Type Conversion6/1
  Bitwise AND2/1 -> Data Type Conversion5/1
  Data Type Conversion4/1 -> Switch1/1
  Data Type Conversion3/1 -> Switch/1
  Delay3/1 -> Switch2/2, Switch1/2, Switch/2, slicing_done/1
  Data Type Conversion5/1 -> Bit Slice4/1, Bit Slice2/1, Bit Slice3/1, Bit Slice1/1, Bit Slice/1
  Bit Slice3/1 -> Bit Concat/2
  Switch/1 -> pos_raw_mt/1, Delay/1
  Bit Slice2/1 -> Bit Concat/3
  Delay/1 -> Switch/3
  Data Type Conversion6/1 -> Switch2/1
  Switch2/1 -> raw_CRC/1, Delay2/1
  Delay2/1 -> Switch2/3

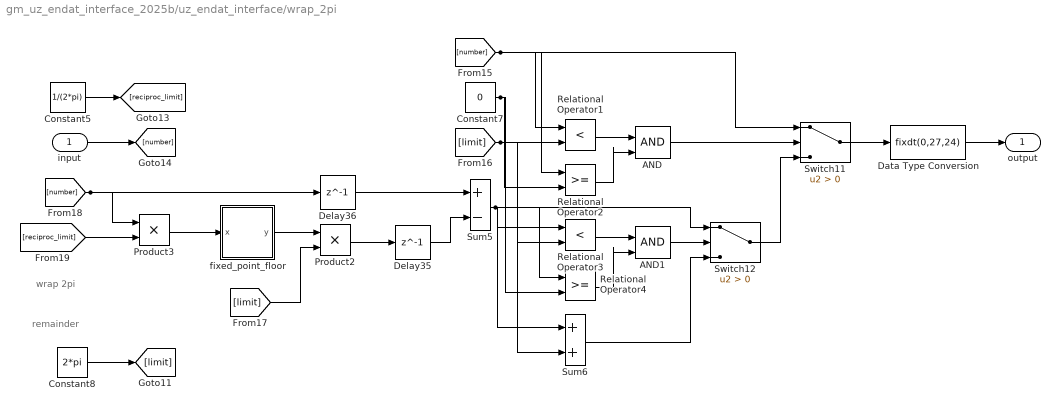
== system gm_uz_endat_interface_2025b/uz_endat_interface/wrap_2pi ==
  note: remainder
  note: wrap 2pi
  input : Inport  OutDataTypeStr=fixdt(0, 27, 20)  PortDimensions=1  SampleTime=1e-08
  AND : Logic  IconShape=distinctive  AllPortsSameDT=off  OutDataTypeStr=boolean
  AND1 : Logic  IconShape=distinctive  AllPortsSameDT=off  OutDataTypeStr=boolean
  Constant5 : Constant  Value=1/(2*pi)  OutDataTypeStr=fixdt(0,18,20)  SampleTime=-1
  Constant7 : Constant  Value=0  OutDataTypeStr=fixdt(0,27,24)  SampleTime=-1
  Constant8 : Constant  Value=2*pi  OutDataTypeStr=fixdt(0,18,15)  SampleTime=-1
  Data Type Conversion : DataTypeConversion  OutDataTypeStr=fixdt(0,27,24)  SaturateOnIntegerOverflow=off  RndMeth=Floor
  Delay35 : Delay  DelayLength=1  InitialCondition=0
  Delay36 : Delay  DelayLength=1  InitialCondition=0
  Product2 : Product  OutDataTypeStr=fixdt(0,27,24)
  Product3 : Product  OutDataTypeStr=fixdt(0,27,24)
  Relational Operator1 : RelationalOperator  Operator=<  OutDataTypeStr=boolean  RndMeth=Simplest  InputSameDT=off
  Relational Operator2 : RelationalOperator  OutDataTypeStr=boolean  RndMeth=Simplest  InputSameDT=off
  Relational Operator3 : RelationalOperator  Operator=<  OutDataTypeStr=boolean  RndMeth=Simplest  InputSameDT=off
  Relational Operator4 : RelationalOperator  OutDataTypeStr=boolean  RndMeth=Simplest  InputSameDT=off
  Sum5 : Sum  Inputs=+-  OutDataTypeStr=fixdt(0,27,24)
  Sum6 : Sum  OutDataTypeStr=fixdt(0,27,24)
  Switch11 : Switch  Criteria=u2 > Threshold  OutDataTypeStr=fixdt(0, 27, 20)  SaturateOnIntegerOverflow=off  InputSameDT=off
  Switch12 : Switch  Criteria=u2 > Threshold  OutDataTypeStr=fixdt(0, 27, 24)  SaturateOnIntegerOverflow=off  InputSameDT=off
  fixed_point_floor : Subsystem
  output : Outport  SampleTime=1e-08
  wires:
  Sum6/1 -> Switch12/3
  Constant5/1 -> [reciproc_limit]
  input/1 -> [number]
  Product3/1 -> fixed_point_floor/1(x)
  Relational Operator2/1 -> AND/2
  Delay36/1 -> Sum5/1
  [number] -> Delay36/1, Product3/1
  Constant8/1 -> [limit]
  [reciproc_limit] -> Product3/2
  [limit] -> Product2/2
  fixed_point_floor/1(y) -> Product2/1
  Product2/1 -> Delay35/1
  Delay35/1 -> Sum5/2
  Relational Operator4/1 -> AND1/2
  [number] -> Switch11/1, Relational Operator2/1, Relational Operator1/1
  Constant7/1 -> Relational Operator4/2, Relational Operator2/2
  [limit] -> Sum6/2, Relational Operator1/2, Relational Operator3/2
  Sum5/1 -> Switch12/1, Relational Operator3/1, Relational Operator4/1, Sum6/1
  Relational Operator1/1 -> AND/1
  Relational Operator3/1 -> AND1/1
  Switch11/1 -> Data Type Conversion/1
  AND/1 -> Switch11/2
  AND1/1 -> Switch12/2
  Switch12/1 -> Switch11/3
  Data Type Conversion/1 -> output/1

== system gm_uz_endat_interface_2025b/uz_endat_interface/position_to_speed_pll/Delay ==
  in0 : Inport  OutDataTypeStr=fixdt(1, 27, 16)  SampleTime=1e-08
  Trigger_emulated : EnablePort  OutDataTypeStr=boolean
  Delay : Delay  DelayLength=double(1)  InitialCondition=0
  out0 : Outport  OutDataTypeStr=fixdt(1, 27, 16)  SampleTime=1e-08  InitialOutput=0
  wires:
  in0/1 -> Delay/1
  Delay/1 -> out0/1

== system gm_uz_endat_interface_2025b/uz_endat_interface/position_to_speed_pll/Delay1 ==
  in0 : Inport  OutDataTypeStr=fixdt(1, 27, 20)  PortDimensions=[2]  SampleTime=1e-08
  Trigger_emulated : EnablePort  OutDataTypeStr=boolean
  Delay1 : Delay  DelayLength=double(1)  InitialCondition=[1 0]
  out0 : Outport  OutDataTypeStr=fixdt(1, 27, 20)  PortDimensions=[2]  SampleTime=1e-08  InitialOutput=0
  wires:
  in0/1 -> Delay1/1
  Delay1/1 -> out0/1

== system gm_uz_endat_interface_2025b/uz_endat_interface/position_to_speed_pll/Delay10 ==
  in0 : Inport  OutDataTypeStr=fixdt(1, 27, 26)  SampleTime=1e-08
  Trigger_emulated : EnablePort  OutDataTypeStr=boolean
  Delay10 : Delay  DelayLength=double(1)  InitialCondition=0
  out0 : Outport  OutDataTypeStr=fixdt(1, 27, 26)  SampleTime=1e-08  InitialOutput=0
  wires:
  in0/1 -> Delay10/1
  Delay10/1 -> out0/1

== system gm_uz_endat_interface_2025b/uz_endat_interface/position_to_speed_pll/Delay11 ==
  in0 : Inport  OutDataTypeStr=fixdt(1, 27, 23)  SampleTime=1e-08
  Trigger_emulated : EnablePort  OutDataTypeStr=boolean
  Delay11 : Delay  DelayLength=double(1)  InitialCondition=0
  out0 : Outport  OutDataTypeStr=fixdt(1, 27, 23)  SampleTime=1e-08  InitialOutput=0
  wires:
  in0/1 -> Delay11/1
  Delay11/1 -> out0/1

== system gm_uz_endat_interface_2025b/uz_endat_interface/position_to_speed_pll/Delay12 ==
  in0 : Inport  OutDataTypeStr=fixdt(1, 27, 20)  SampleTime=1e-08
  Trigger_emulated : EnablePort  OutDataTypeStr=boolean
  Delay12 : Delay  DelayLength=double(1)  InitialCondition=0
  out0 : Outport  OutDataTypeStr=fixdt(1, 27, 20)  SampleTime=1e-08  InitialOutput=0
  wires:
  in0/1 -> Delay12/1
  Delay12/1 -> out0/1

== system gm_uz_endat_interface_2025b/uz_endat_interface/position_to_speed_pll/Delay13 ==
  in0 : Inport  OutDataTypeStr=fixdt(0, 27, 24)  SampleTime=1e-08
  Trigger_emulated : EnablePort  OutDataTypeStr=boolean
  Delay13 : Delay  DelayLength=double(1)  InitialCondition=0
  out0 : Outport  OutDataTypeStr=fixdt(0, 27, 24)  SampleTime=1e-08  InitialOutput=0
  wires:
  in0/1 -> Delay13/1
  Delay13/1 -> out0/1

== system gm_uz_endat_interface_2025b/uz_endat_interface/position_to_speed_pll/Delay14 ==
  in0 : Inport  OutDataTypeStr=fixdt(1, 27, 20)  SampleTime=1e-08
  Trigger_emulated : EnablePort  OutDataTypeStr=boolean
  Delay14 : Delay  DelayLength=double(1)  InitialCondition=0
  out0 : Outport  OutDataTypeStr=fixdt(1, 27, 20)  SampleTime=1e-08  InitialOutput=0
  wires:
  in0/1 -> Delay14/1
  Delay14/1 -> out0/1

== system gm_uz_endat_interface_2025b/uz_endat_interface/position_to_speed_pll/Delay18 ==
  in0 : Inport  OutDataTypeStr=fixdt(1, 27, 20)  PortDimensions=[2]  SampleTime=1e-08
  Trigger_emulated : EnablePort  OutDataTypeStr=boolean
  Delay18 : Delay  DelayLength=double(1)  InitialCondition=[1 0]
  out0 : Outport  OutDataTypeStr=fixdt(1, 27, 20)  PortDimensions=[2]  SampleTime=1e-08  InitialOutput=0
  wires:
  in0/1 -> Delay18/1
  Delay18/1 -> out0/1

== system gm_uz_endat_interface_2025b/uz_endat_interface/position_to_speed_pll/Delay19 ==
  in0 : Inport  OutDataTypeStr=fixdt(1, 27, 23)  SampleTime=1e-08
  Trigger_emulated : EnablePort  OutDataTypeStr=boolean
  Delay19 : Delay  DelayLength=double(1)  InitialCondition=0
  out0 : Outport  OutDataTypeStr=fixdt(1, 27, 23)  SampleTime=1e-08  InitialOutput=0
  wires:
  in0/1 -> Delay19/1
  Delay19/1 -> out0/1

== system gm_uz_endat_interface_2025b/uz_endat_interface/position_to_speed_pll/Delay2 ==
  in0 : Inport  OutDataTypeStr=fixdt(1, 27, 24)  SampleTime=1e-08
  Trigger_emulated : EnablePort  OutDataTypeStr=boolean
  Delay2 : Delay  DelayLength=double(1)  InitialCondition=0
  out0 : Outport  OutDataTypeStr=fixdt(1, 27, 24)  SampleTime=1e-08  InitialOutput=0
  wires:
  in0/1 -> Delay2/1
  Delay2/1 -> out0/1

== system gm_uz_endat_interface_2025b/uz_endat_interface/position_to_speed_pll/Delay20 ==
  in0 : Inport  OutDataTypeStr=boolean  SampleTime=1e-08
  Trigger_emulated : EnablePort  OutDataTypeStr=boolean
  Delay20 : Delay  DelayLength=double(1)  InitialCondition=0
  out0 : Outport  OutDataTypeStr=boolean  SampleTime=1e-08  InitialOutput=0
  wires:
  in0/1 -> Delay20/1
  Delay20/1 -> out0/1

== system gm_uz_endat_interface_2025b/uz_endat_interface/position_to_speed_pll/Delay21 ==
  in0 : Inport  OutDataTypeStr=boolean  SampleTime=1e-08
  Trigger_emulated : EnablePort  OutDataTypeStr=boolean
  Delay21 : Delay  DelayLength=double(1)  InitialCondition=0
  out0 : Outport  OutDataTypeStr=boolean  SampleTime=1e-08  InitialOutput=0
  wires:
  in0/1 -> Delay21/1
  Delay21/1 -> out0/1

== system gm_uz_endat_interface_2025b/uz_endat_interface/position_to_speed_pll/Delay22 ==
  in0 : Inport  OutDataTypeStr=fixdt(1, 27, 20)  SampleTime=1e-08
  Trigger_emulated : EnablePort  OutDataTypeStr=boolean
  Delay22 : Delay  DelayLength=double(1)  InitialCondition=0
  out0 : Outport  OutDataTypeStr=fixdt(1, 27, 20)  SampleTime=1e-08  InitialOutput=0
  wires:
  in0/1 -> Delay22/1
  Delay22/1 -> out0/1

== system gm_uz_endat_interface_2025b/uz_endat_interface/position_to_speed_pll/Delay23 ==
  in0 : Inport  OutDataTypeStr=fixdt(1, 27, 20)  SampleTime=1e-08
  Trigger_emulated : EnablePort  OutDataTypeStr=boolean
  Delay23 : Delay  DelayLength=double(1)  InitialCondition=0
  out0 : Outport  OutDataTypeStr=fixdt(1, 27, 20)  SampleTime=1e-08  InitialOutput=0
  wires:
  in0/1 -> Delay23/1
  Delay23/1 -> out0/1

== system gm_uz_endat_interface_2025b/uz_endat_interface/position_to_speed_pll/Delay3 ==
  in0 : Inport  OutDataTypeStr=fixdt(1, 27, 14)  SampleTime=1e-08
  Trigger_emulated : EnablePort  OutDataTypeStr=boolean
  Delay3 : Delay  DelayLength=double(1)  InitialCondition=0
  out0 : Outport  OutDataTypeStr=fixdt(1, 27, 14)  SampleTime=1e-08  InitialOutput=0
  wires:
  in0/1 -> Delay3/1
  Delay3/1 -> out0/1

== system gm_uz_endat_interface_2025b/uz_endat_interface/position_to_speed_pll/Delay4 ==
  in0 : Inport  OutDataTypeStr=fixdt(1, 27, 20)  SampleTime=1e-08
  Trigger_emulated : EnablePort  OutDataTypeStr=boolean
  Delay4 : Delay  DelayLength=double(1)  InitialCondition=0
  out0 : Outport  OutDataTypeStr=fixdt(1, 27, 20)  SampleTime=1e-08  InitialOutput=0
  wires:
  in0/1 -> Delay4/1
  Delay4/1 -> out0/1

== system gm_uz_endat_interface_2025b/uz_endat_interface/position_to_speed_pll/Delay5 ==
  in0 : Inport  OutDataTypeStr=fixdt(1, 27, 8)  SampleTime=1e-08
  Trigger_emulated : EnablePort  OutDataTypeStr=boolean
  Delay5 : Delay  DelayLength=double(1)  InitialCondition=0
  out0 : Outport  OutDataTypeStr=fixdt(1, 27, 8)  SampleTime=1e-08  InitialOutput=0
  wires:
  in0/1 -> Delay5/1
  Delay5/1 -> out0/1

== system gm_uz_endat_interface_2025b/uz_endat_interface/position_to_speed_pll/Delay6 ==
  in0 : Inport  OutDataTypeStr=fixdt(0, 18, 24)  SampleTime=1e-08
  Trigger_emulated : EnablePort  OutDataTypeStr=boolean
  Delay6 : Delay  DelayLength=double(1)  InitialCondition=0
  out0 : Outport  OutDataTypeStr=fixdt(0, 18, 24)  SampleTime=1e-08  InitialOutput=0
  wires:
  in0/1 -> Delay6/1
  Delay6/1 -> out0/1

== system gm_uz_endat_interface_2025b/uz_endat_interface/position_to_speed_pll/Delay7 ==
  in0 : Inport  OutDataTypeStr=fixdt(0, 18, 0)  SampleTime=1e-08
  Trigger_emulated : EnablePort  OutDataTypeStr=boolean
  Delay7 : Delay  DelayLength=double(1)  InitialCondition=0
  out0 : Outport  OutDataTypeStr=fixdt(0, 18, 0)  SampleTime=1e-08  InitialOutput=0
  wires:
  in0/1 -> Delay7/1
  Delay7/1 -> out0/1

== system gm_uz_endat_interface_2025b/uz_endat_interface/position_to_speed_pll/Delay8 ==
  in0 : Inport  OutDataTypeStr=fixdt(0, 18, 5)  SampleTime=1e-08
  Trigger_emulated : EnablePort  OutDataTypeStr=boolean
  Delay8 : Delay  DelayLength=double(1)  InitialCondition=0
  out0 : Outport  OutDataTypeStr=fixdt(0, 18, 5)  SampleTime=1e-08  InitialOutput=0
  wires:
  in0/1 -> Delay8/1
  Delay8/1 -> out0/1

== system gm_uz_endat_interface_2025b/uz_endat_interface/position_to_speed_pll/Delay9 ==
  in0 : Inport  OutDataTypeStr=fixdt(1, 27, 14)  SampleTime=1e-08
  Trigger_emulated : EnablePort  OutDataTypeStr=boolean
  Delay9 : Delay  DelayLength=double(1)  InitialCondition=0
  out0 : Outport  OutDataTypeStr=fixdt(1, 27, 14)  SampleTime=1e-08  InitialOutput=0
  wires:
  in0/1 -> Delay9/1
  Delay9/1 -> out0/1

== system gm_uz_endat_interface_2025b/uz_endat_interface/position_to_speed_pll/Sine HDL Optimized ==
  u : Inport  OutDataTypeStr=fixdt(1, 27, 20)  SampleTime=1e-08
  sincos hdl : Subsystem  mask{NumDataPoints=256, TableDataTypeStr=fixdt(0,26,20), SimulateLUTROMDelay='Off'}
      mask prompts: NumDataPoints "HDLShared:hdlshared:CosineHDL_Npts"; TableDataTypeStr "Simulink:blkprm_prompts:TABLE_UNIFIEDDATATYPE"; SimulateLUTROMDelay "HDLShared:hdlshared:CosineHDL_SimulateLUTDelay"
      mask Display:
      | port_label('input',1,'u')
      | port_label('output',1,'sin(2*pi*u)')
      | port_label('output',2,'cos(2*pi*u)')
      | xpos = 0.35;
      | yoffset = 0.5;
      | if ( SimulateLUTROMDelay )
      |   text(xpos,yoffset,'HDL (Z^{-1})','texmode','on')
      | else
      |    text(xpos,yoffset,'HDL')
      | end
  x : Outport  SampleTime=1e-08  VectorParamsAs1DForOutWhenUnconnected=off
  y : Outport  Port=2  SampleTime=1e-08
  wires:
  u/1 -> sincos hdl/1(In1)
  sincos hdl/1(Out1) -> x/1
  sincos hdl/2(Out2) -> y/1
